simulink model "exampleMaxRunTime"  (Simulink 7.6)
settings: Solver=ode45  StartTime=0.0  StopTime=30  RelTol=1e-3
settings Model: Creator=drhf  LastModifiedBy=awohlfei
settings CodeAppCC: CustomSymbolStrType=$N$R$M_T

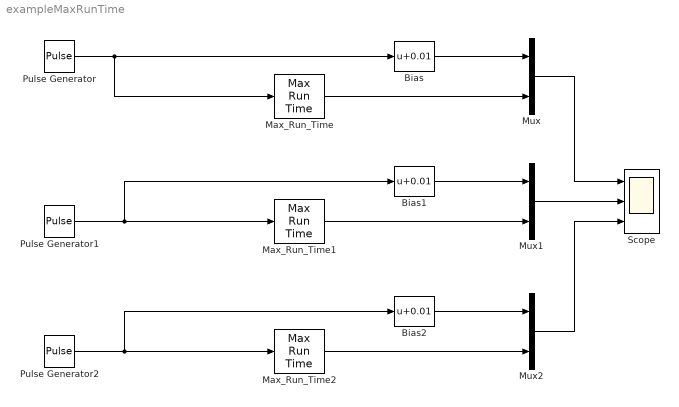
== system exampleMaxRunTime ==
  Bias : Bias  Bias=0.01
  Bias1 : Bias  Bias=0.01
  Bias2 : Bias  Bias=0.01
  Max_Run_Time : Reference  SystemSampleTime=-1  tmaxrun=5
  Max_Run_Time1 : Reference  SystemSampleTime=-1  tmaxrun=5
  Max_Run_Time2 : Reference  SystemSampleTime=-1  tmaxrun=5
  Mux : Mux  Inputs=2
  Mux1 : Mux  Inputs=2
  Mux2 : Mux  Inputs=2
  Pulse Generator : DiscretePulseGenerator  PulseType=Time based  Amplitude=2  Period=10  PulseWidth=80
  Pulse Generator1 : DiscretePulseGenerator  PulseType=Time based  Amplitude=2  Period=10  PulseWidth=10
  Pulse Generator2 : DiscretePulseGenerator  PulseType=Time based  Amplitude=2  Period=20  PulseWidth=90
  Scope : Scope  NumInputPorts=3
      settings: YMin=-5~-5~-5  YMax=5~5~5
  wires:
  Pulse Generator/1 -> Max_Run_Time/1, Bias/1
  Mux/1 -> Scope/1
  Max_Run_Time/1 -> Mux/2
  Pulse Generator1/1 -> Max_Run_Time1/1, Bias1/1
  Max_Run_Time1/1 -> Mux1/2
  Mux1/1 -> Scope/2
  Bias/1 -> Mux/1
  Bias1/1 -> Mux1/1
  Pulse Generator2/1 -> Bias2/1, Max_Run_Time2/1
  Max_Run_Time2/1 -> Mux2/2
  Mux2/1 -> Scope/3
  Bias2/1 -> Mux2/1
